simulink model "testmdl1"  (R2016b)
settings: Solver=VariableStepAuto  StartTime=0.0  StopTime=10.0  RelTol=1e-3
settings Model: Creator=sgopalswamy  LastModifiedBy=sgopalswamy
settings DataIOCC: LimitDataPoints=on  SaveOutput=off  SaveTime=off
settings OptimizationCC: BlockReduction=off  BooleanDataType=off  LifeSpan=inf
settings DebuggingCC: SaveWithParameterizedLinksMsg=none  UnderspecifiedInitializationDetection=Classic  MergeDetectMultiDrivingBlocksExec=none  SignalResolutionControl=TryResolveAllWithWarning  AllowSymbolicDim=off  SFUnexpectedBacktrackingDiag=warning  SFNoUnconditionalDefaultTransitionDiag=warning  SFExecutionAtInitializationDiag=none
settings HardwareCC: TargetUnknown=on
settings GRTTargetCC: TargetLangStandard=C89/C90 (ANSI)  GeneratePreprocessorConditionals=Disable all

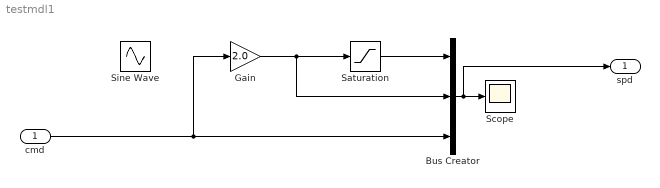
== system testmdl1 ==
  cmd : Inport
  Bus Creator : BusCreator  Inputs=3
  Gain : Gain  Gain=2.0
  Saturation : Saturate
  Scope : Scope
  Sine Wave : Sin  SampleTime=0
  spd : Outport
  wires:
  Gain/1 -> Bus Creator/2, Saturation/1
  Bus Creator/1 -> spd/1, Scope/1
  Saturation/1 -> Bus Creator/1
  cmd/1 -> Bus Creator/3, Gain/1
